simulink model "chap7_1sim"  (Simulink 6.3)
settings: Solver=ode45  StartTime=0.0  StopTime=100  FixedStep=0.001  RelTol=1e-3
settings Model: Creator=hp  LastModifiedBy=Administrator  ExtModeTrigMode=oneshot  ExtModeArmWhenConnect=off
settings DataIOCC: LimitDataPoints=off  SignalLoggingName=sigsOut
settings OptimizationCC: BooleanDataType=off
settings DebuggingCC: SolverPrmCheckMsg=none
settings HardwareCC: TargetUnknown=on

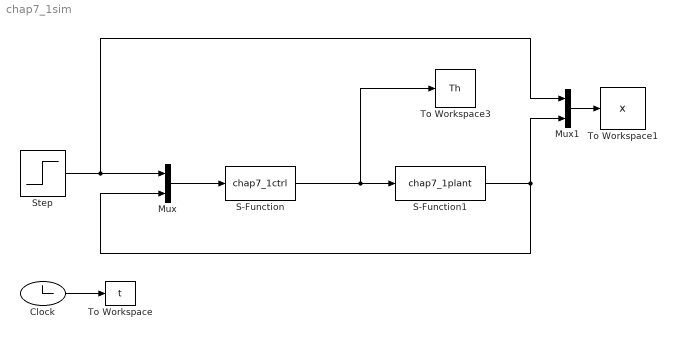
== system chap7_1sim ==
  Clock : Clock
  Mux : Mux  Inputs=2
  Mux1 : Mux  Inputs=2
  S-Function : S-Function  FunctionName=chap7_1ctrl
  S-Function1 : S-Function  FunctionName=chap7_1plant
  Step : Step  Time=0  After=pi/3  SampleTime=0
  To Workspace : ToWorkspace  VariableName=t  SampleTime=-1  SaveFormat=Array
  To Workspace1 : ToWorkspace  VariableName=x  SampleTime=-1  SaveFormat=Array
  To Workspace3 : ToWorkspace  VariableName=Th  SampleTime=-1  SaveFormat=Array
  wires:
  Clock/1 -> To Workspace/1
  Step/1 -> Mux/1, Mux1/1
  Mux1/1 -> To Workspace1/1
  Mux/1 -> S-Function/1
  S-Function1/1 -> Mux/2, Mux1/2
  S-Function/1 -> To Workspace3/1, S-Function1/1
